simulink model "Motores"  (R2023b)
settings: Solver=VariableStepAuto  StartTime=0.0  StopTime=10.0  RelTol=1e-3
libraries: arduinolib x6
settings Model: Creator=Daniel  LastModifiedBy=Daniel

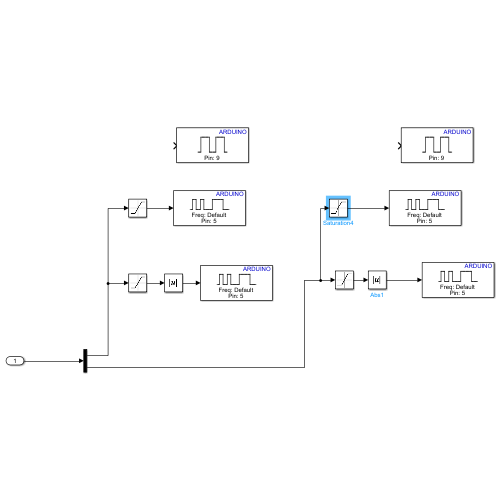
[thumbnail: Simulink's stored preview of the top-level diagram]
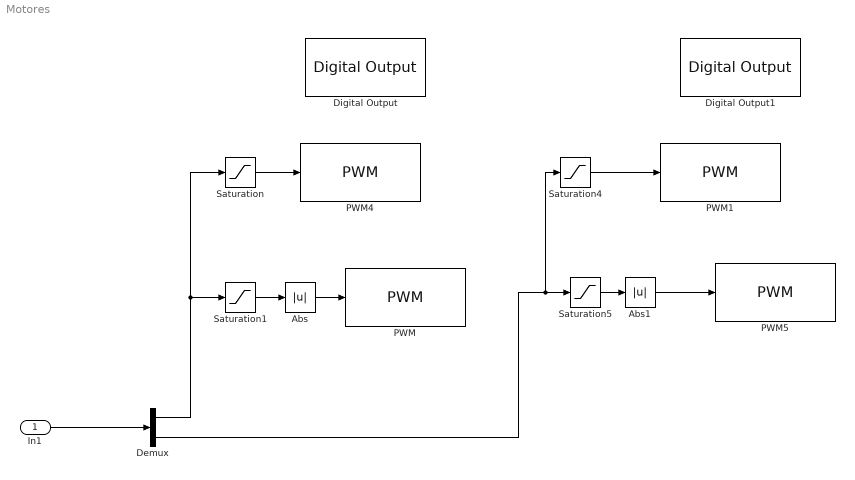
== system Motores ==
  In1 : Inport
  Abs : Abs  SaturateOnIntegerOverflow=off
  Abs1 : Abs  SaturateOnIntegerOverflow=off
  Demux : Demux  Outputs=2
  Digital Output : arduinolib/Digital Output  pinNumber=9  Direction=output  blockPlatform=arduino
  Digital Output1 : arduinolib/Digital Output  pinNumber=9  Direction=output  blockPlatform=arduino
  PWM{,1,4..5} (4 alike) : arduinolib/PWM  pinNumber=5  frequencyType=Default  desiredFrequency=490.2  achievableFrequency=490.2
  Saturation{,1,4..5} (4 alike) : Saturate  UpperLimit=255  LowerLimit=0
  wires:
  Saturation1/1 -> Abs/1
  Saturation5/1 -> Abs1/1
  In1/1 -> Demux/1
  Abs/1 -> PWM/1
  Saturation/1 -> PWM4/1
  Saturation4/1 -> PWM1/1
  Abs1/1 -> PWM5/1
  Demux/2 -> Saturation4/1, Saturation5/1
  Demux/1 -> Saturation/1, Saturation1/1
